simulink model "Registro_TEST_a"  (R2020a)
settings: Solver=VariableStepAuto  StartTime=0.0  StopTime=40  RelTol=1e-3
settings Model: DataDictionary=Registro_variables.sldd  Creator=Juan  LastModifiedBy=Juan

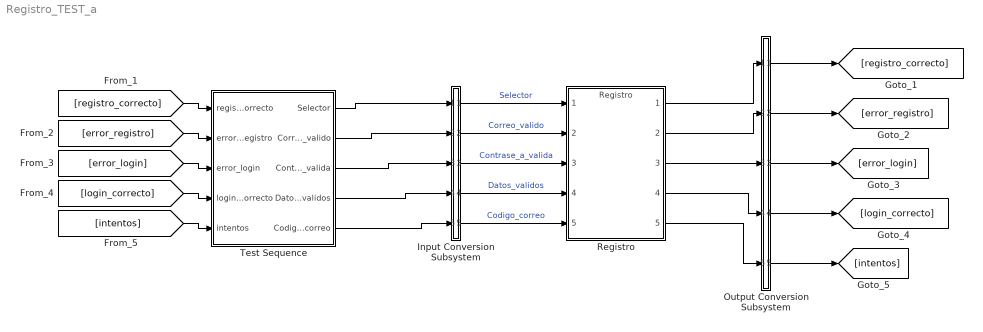
== system Registro_TEST_a ==
  Input Conversion Subsystem : Subsystem  Tag=__SLT_ICS__  Description=|
      | Signal spec.
      | and routing
      settings: AttributesFormatString=%<Description>
  Output Conversion Subsystem : Subsystem  Tag=__SLT_OCS__  Description=|
      | Signal spec.
      | and routing
      settings: AttributesFormatString=%<Description>
  Registro : ModelReference  ModelNameDialog=Registro  SimulationMode=Normal  ModelReferenceVersion=1.58
  Test Sequence : Test Sequence  TreatAsAtomicUnit=on
  wires:
  Test Sequence/1(Selector) -> Input Conversion Subsystem/1(Inport_1)
  Test Sequence/2(Correo_valido) -> Input Conversion Subsystem/2(Inport_2)
  Test Sequence/3(Contrase_a_valida) -> Input Conversion Subsystem/3(Inport_3)
  Test Sequence/4(Datos_validos) -> Input Conversion Subsystem/4(Inport_4)
  Test Sequence/5(Codigo_correo) -> Input Conversion Subsystem/5(Inport_5)
  [registro_correcto] -> Test Sequence/1(registro_correcto)
  [error_registro] -> Test Sequence/2(error_registro)
  [error_login] -> Test Sequence/3(error_login)
  [login_correcto] -> Test Sequence/4(login_correcto)
  [intentos] -> Test Sequence/5(intentos)
  Output Conversion Subsystem/1(Outport_1) -> [registro_correcto]
  Output Conversion Subsystem/2(Outport_2) -> [error_registro]
  Output Conversion Subsystem/3(Outport_3) -> [error_login]
  Output Conversion Subsystem/4(Outport_4) -> [login_correcto]
  Output Conversion Subsystem/5(Outport_5) -> [intentos]
  Input Conversion Subsystem/1(Outport_1) -> Registro/1  "Selector"
  Input Conversion Subsystem/2(Outport_2) -> Registro/2  "Correo_valido"
  Input Conversion Subsystem/3(Outport_3) -> Registro/3  "Contrase_a_valida"
  Input Conversion Subsystem/4(Outport_4) -> Registro/4  "Datos_validos"
  Input Conversion Subsystem/5(Outport_5) -> Registro/5  "Codigo_correo"
  Registro/1 -> Output Conversion Subsystem/1(Inport_1)
  Registro/2 -> Output Conversion Subsystem/2(Inport_2)
  Registro/3 -> Output Conversion Subsystem/3(Inport_3)
  Registro/4 -> Output Conversion Subsystem/4(Inport_4)
  Registro/5 -> Output Conversion Subsystem/5(Inport_5)

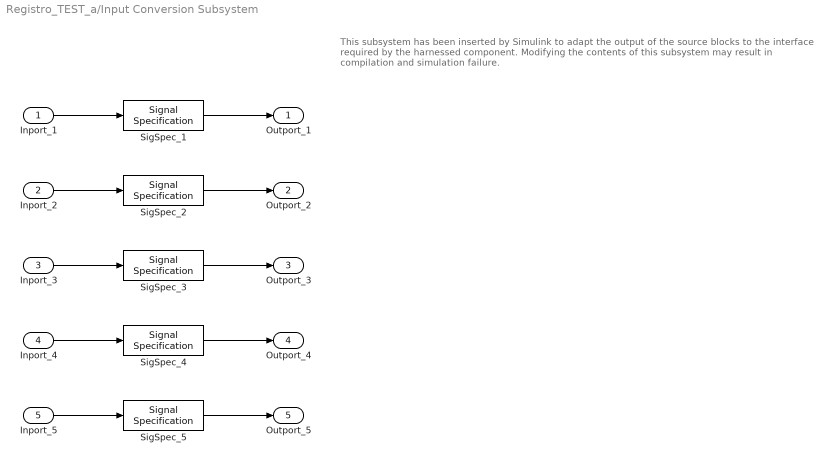
== system Registro_TEST_a/Input Conversion Subsystem ==
  note: This subsystem has been inserted by Simulink to adapt the output of the source blocks to the interface required by the harnessed component.
      |  Modifying the contents of this subsystem may result in compilation and simulation failure.
  Inport_1 : Inport
  Inport_2 : Inport  Port=2
  Inport_3 : Inport  Port=3
  Inport_4 : Inport  Port=4
  Inport_5 : Inport  Port=5
  SigSpec_1 : SignalSpecification  OutDataTypeStr=double  Dimensions=[1]  SampleTime=[-1, 0]
  SigSpec_{2..5} (4 alike) : SignalSpecification  OutDataTypeStr=boolean  Dimensions=[1]  SampleTime=[-1, 0]
  Outport_1 : Outport
  Outport_2 : Outport  Port=2
  Outport_3 : Outport  Port=3
  Outport_4 : Outport  Port=4
  Outport_5 : Outport  Port=5
  wires:
  SigSpec_1/1 -> Outport_1/1
  Inport_1/1 -> SigSpec_1/1
  SigSpec_2/1 -> Outport_2/1
  Inport_2/1 -> SigSpec_2/1
  SigSpec_3/1 -> Outport_3/1
  Inport_3/1 -> SigSpec_3/1
  SigSpec_4/1 -> Outport_4/1
  Inport_4/1 -> SigSpec_4/1
  SigSpec_5/1 -> Outport_5/1
  Inport_5/1 -> SigSpec_5/1

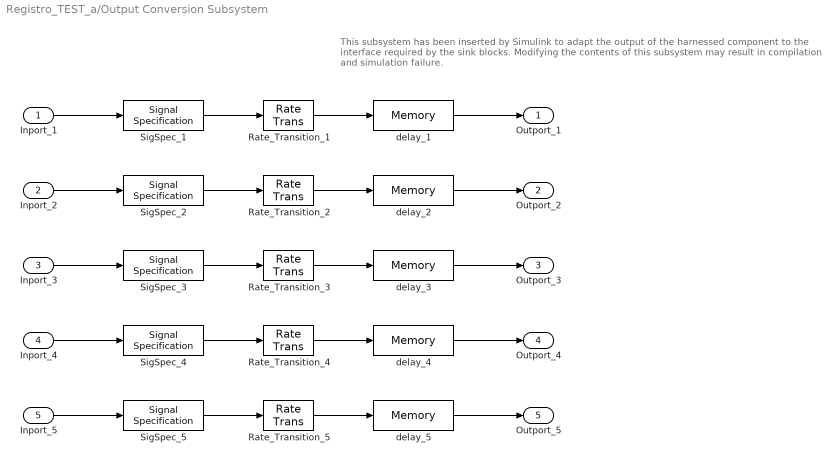
== system Registro_TEST_a/Output Conversion Subsystem ==
  note: This subsystem has been inserted by Simulink to adapt the output of the harnessed component to the interface required by the sink blocks.
      |  Modifying the contents of this subsystem may result in compilation and simulation failure.
  Inport_1 : Inport
  Inport_2 : Inport  Port=2
  Inport_3 : Inport  Port=3
  Inport_4 : Inport  Port=4
  Inport_5 : Inport  Port=5
  Rate_Transition_{1..5} (5 alike) : RateTransition  OutPortSampleTimeOpt=Inherit
  SigSpec_{1..4} (4 alike) : SignalSpecification  OutDataTypeStr=boolean  Dimensions=[1]
  SigSpec_5 : SignalSpecification  OutDataTypeStr=double  Dimensions=[1]
  delay_{1..5} (5 alike) : Memory
  Outport_1 : Outport
  Outport_2 : Outport  Port=2
  Outport_3 : Outport  Port=3
  Outport_4 : Outport  Port=4
  Outport_5 : Outport  Port=5
  wires:
  Inport_1/1 -> SigSpec_1/1
  SigSpec_1/1 -> Rate_Transition_1/1
  Rate_Transition_1/1 -> delay_1/1
  delay_1/1 -> Outport_1/1
  Inport_2/1 -> SigSpec_2/1
  SigSpec_2/1 -> Rate_Transition_2/1
  Rate_Transition_2/1 -> delay_2/1
  delay_2/1 -> Outport_2/1
  Inport_3/1 -> SigSpec_3/1
  SigSpec_3/1 -> Rate_Transition_3/1
  Rate_Transition_3/1 -> delay_3/1
  delay_3/1 -> Outport_3/1
  Inport_4/1 -> SigSpec_4/1
  SigSpec_4/1 -> Rate_Transition_4/1
  Rate_Transition_4/1 -> delay_4/1
  delay_4/1 -> Outport_4/1
  Inport_5/1 -> SigSpec_5/1
  SigSpec_5/1 -> Rate_Transition_5/1
  Rate_Transition_5/1 -> delay_5/1
  delay_5/1 -> Outport_5/1

== stateflow chart Registro_TEST_a/Test Sequence ==
  settings: stateMachineType=SIMPLIFIED_MACHINE
  state Run
    %% Initialize data outputs.
    Selector = 0;
    Correo_valido = false;
    Contrase_a_valida = false;
    Datos_validos = false;
    Codigo_correo = false;
  state step_1
    Selector = 1;
  state step_2
    Correo_valido = true;
  state step_3
    Contrase_a_valida = true;
  state step_4
    Datos_validos = true;
  state step_5
    Codigo_correo = true;
    Selector = 2
  state step_6
    Correo_valido = false;
    Contrase_a_valida = false;
    Datos_validos = false;
    Codigo_correo = false;
    if(login_correcto)
    Selector = 0
    end
  state step_7
    Selector = 0;
  (default) -> Run
  Run -> step_1 : [
      | after(1,msec)
      | ]
  step_1 -> step_2 : [
      | after(1,sec)
      | ]
  (junction 70) -> step_2
  (junction 72) -> (junction 70)
  step_2 -> step_3 : [
      | after(1,sec)
      | ]
  step_3 -> step_4 : [
      | after(1,sec)
      | ]
  step_4 -> step_5 : [
      | after(1,sec)
      | ]
  step_5 -> step_6 : [
      | after(1,sec)
      | ]
  step_6 -> (junction 72) [order 1] : [
      | after(1,sec)
      | ]
  step_6 -> step_7 [order 2] : [
      | Selector == 0
      | ]
  data: registro_correcto input boolean size=[1]; error_registro input boolean size=[1]; error_login input boolean size=[1]; login_correcto input boolean size=[1]; intentos input double size=[1]; Selector output double size=[1]; Correo_valido output boolean size=[1]; Contrase_a_valida output boolean size=[1]; Datos_validos output boolean size=[1]; Codigo_correo output boolean size=[1]
